simulink model "PIDwirnik"  (R2015a)
settings: Solver=ode3  StartTime=0.0  StopTime=10  FixedStep=0.02  RelTol=1e-3
values from neighbouring files (symbols this model uses):
  B = 0.5    [wirnik.m]    (also in wirnik1.m)
  J = 0.01    [SilnikDC.m]    (also in funkcja.m; modelmplik.m; wirnik.m = 0.1; wirnik1.m = 0.1)
  Kd = output(2)    [SilnikDC.m]    (also in funkcja.m = pid(2); funkcja1.m = pid(3); grzalka.m = output(3); grzałka.m = output(3))
  ke = 0.1    [wirnik.m]    (also in wirnik1.m = 1)
  Ki = output(3)    [SilnikDC.m]    (also in funkcja.m = pid(3); funkcja1.m = pid(2); grzalka.m = output(2); grzałka.m = output(2))
  km = 0.1    [wirnik.m]    (also in wirnik1.m)
  Kp = output(1)    [SilnikDC.m]    (also in funkcja.m = pid(1); funkcja1.m = pid(1); grzalka.m; grzałka.m)
  Lw = 2.0    (= 2)    [wirnik.m]    (also in wirnik1.m)
  Rw = 2.0    (= 2)    [wirnik.m]    (also in wirnik1.m)
settings Model: Creator=Dawid  LastModifiedBy=Dawid

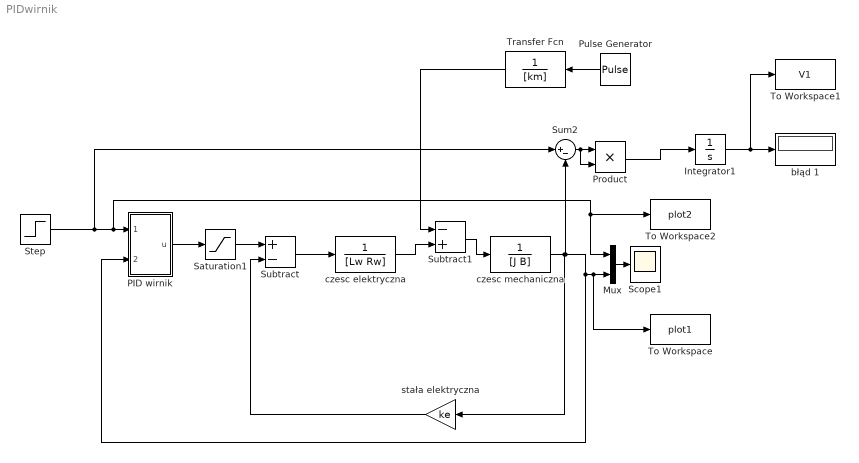
== system PIDwirnik ==
  Integrator1 : Integrator
  Mux : Mux  Inputs=2
  "PID wirnik " : Subsystem
  Product : Product
  Pulse Generator : DiscretePulseGenerator  PulseType=Time based  Amplitude=0.2  PulseWidth=10
  Saturation1 : Saturate  UpperLimit=300  LowerLimit=-300  ZeroCross=off
  Scope1 : Scope
  Step : Step  Time=0  SampleTime=0.02
  Subtract : Sum  Inputs=+-
  Subtract1 : Sum  Inputs=-+
  Sum2 : Sum  Inputs=|+-
  To Workspace : ToWorkspace  VariableName=plot1  SaveFormat=Structure With Time  SampleTime=-1
  To Workspace1 : ToWorkspace  VariableName=V1  SampleTime=-1
  To Workspace2 : ToWorkspace  VariableName=plot2  SaveFormat=Structure With Time  SampleTime=-1
  Transfer Fcn : TransferFcn  Denominator=[km]
  błąd 1 : Display
  "czesc elektryczna " : TransferFcn  Denominator=[Lw Rw]
  "czesc mechaniczna " : TransferFcn  Denominator=[J B]
  "stała elektryczna " : Gain  Gain=ke
  wires:
  Integrator1/1 -> To Workspace1/1, błąd 1/1
  Subtract1/1 -> "czesc mechaniczna "/1
  "stała elektryczna "/1 -> Subtract/2
  Subtract/1 -> "czesc elektryczna "/1
  Step/1 -> Sum2/1, To Workspace2/1, Mux/1, "PID wirnik "/1("1 ")
  "PID wirnik "/1(u) -> Saturation1/1
  "czesc mechaniczna "/1 -> "stała elektryczna "/1, To Workspace/1, Mux/2, "PID wirnik "/2(2), Sum2/2
  Saturation1/1 -> Subtract/1
  Mux/1 -> Scope1/1
  "czesc elektryczna "/1 -> Subtract1/2
  Product/1 -> Integrator1/1
  Pulse Generator/1 -> Transfer Fcn/1
  Transfer Fcn/1 -> Subtract1/1
  Sum2/1 -> Product/2, Product/1

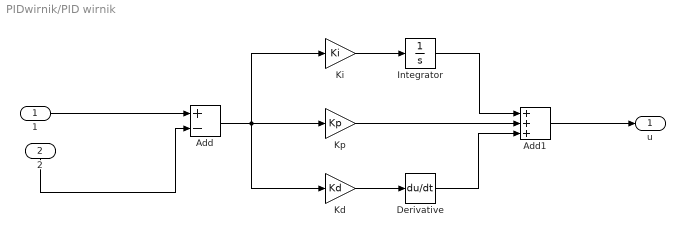
== system PIDwirnik/PID wirnik  ==
  "1 " : Inport
  2 : Inport  Port=2
  Add : Sum  Inputs=+-
  Add1 : Sum  Inputs=+++
  Derivative : Derivative
  Integrator : Integrator
  Kd : Gain  Gain=Kd
  "Ki " : Gain  Gain=Ki
  Kp : Gain  Gain=Kp
  u : Outport
  wires:
  Kp/1 -> Add1/2
  Integrator/1 -> Add1/1
  Kd/1 -> Derivative/1
  "Ki "/1 -> Integrator/1
  Add/1 -> Kd/1, "Ki "/1, Kp/1
  Add1/1 -> u/1
  Derivative/1 -> Add1/3
  "1 "/1 -> Add/1
  2/1 -> Add/2
